simulink model "MPC_Cotroller_ahi"  (R2023a)
settings: Solver=FixedStepAuto  StartTime=0.0  StopTime=10  FixedStep=0.02  RelTol=1e-3
settings Model: Creator=NEW  LastModifiedBy=NEW
settings DebuggingCC: UnderSpecifiedDimensionMsg=warning

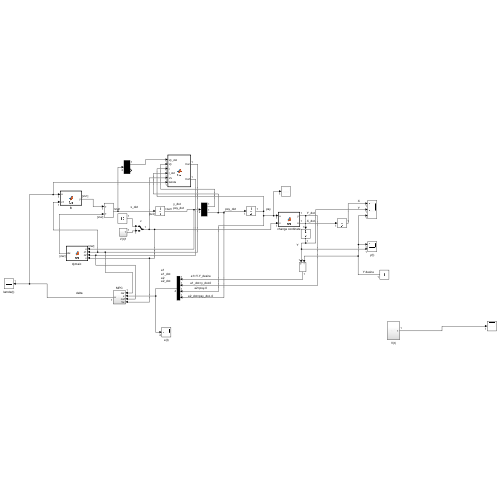
[thumbnail: Simulink's stored preview of the top-level diagram]
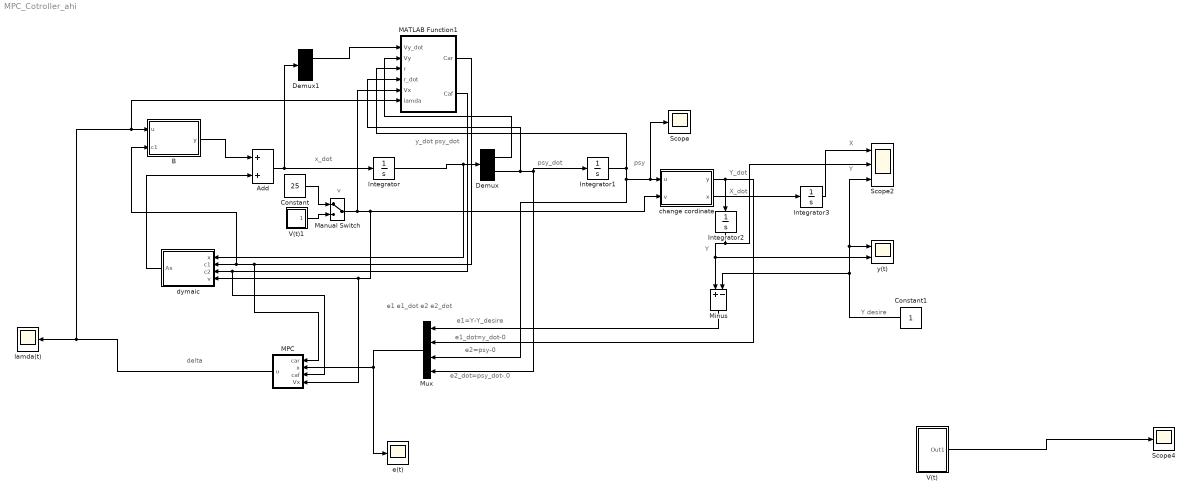
== system MPC_Cotroller_ahi ==
  note: X
  note: X_dot
  note: delta
  note: v
  note: e1
      | e1_dot
      | e2
      | e2_dot
  note: e2_dot=psy_dot-.0
  note: e2=psy-0
  note: e1_dot=y_dot-0
  note: e1=Y-Y_desire
  note: Y desire
  note: Y
  note: Y_dot
  note: psy
  note: psy_dot
  note: y_dot
      | psy_dot
  note: x_dot
  note: Y
  Add : Sum
  B : MATLAB Function  TreatAsAtomicUnit=on
  Constant : Constant  Value=25
  Constant1 : Constant
  Demux : Demux  Outputs=2
  Demux1 : Demux  Outputs=2
  Integrator{,1..3} (4 alike) : Integrator
  MATLAB Function1 : MATLAB Function  TreatAsAtomicUnit=on
  MPC : Subsystem
  Manual Switch : ManualSwitch
  Minus : Sum  Inputs=+-
  Mux : Mux
  Scope : Scope
  Scope2 : Scope  NumInputPorts=3
  Scope4 : Scope
  V(t) : Subsystem
  V(t)1 : Subsystem
  change cordinate : MATLAB Function  TreatAsAtomicUnit=on
  "dymaic " : MATLAB Function  TreatAsAtomicUnit=on
  e(t) : Scope
  lamda(t) : Scope
  y(t) : Scope  NumInputPorts=2
  wires:
  Integrator/1 -> "dymaic "/1(x), Demux/1
  "dymaic "/1(Ax) -> Add/2
  Integrator1/1 -> Mux/3, Scope/1, change cordinate/1(u), MATLAB Function1/3(r)
  Demux/2 -> MATLAB Function1/4(r_dot), Mux/4, Integrator1/1
  change cordinate/1(y) -> Integrator2/1, Mux/2
  Integrator2/1 -> y(t)/2, Minus/1, Scope2/2
  Minus/1 -> Mux/1
  Mux/1 -> e(t)/1, MPC/2(x)
  MPC/1(u) -> MATLAB Function1/6(lamda), B/1(u), lamda(t)/1
  B/1(y) -> Add/1
  Manual Switch/1 -> MATLAB Function1/5(Vx), "dymaic "/4(v), MPC/4(Vx), change cordinate/2(v)
  V(t)/1(Out1) -> Scope4/1
  Constant/1 -> Manual Switch/1
  V(t)1/1(Out1) -> Manual Switch/2
  Integrator3/1 -> Scope2/1
  change cordinate/2(x) -> Integrator3/1
  Constant1/1 -> Scope2/3, y(t)/1, Minus/2
  Add/1 -> Integrator/1, Demux1/1
  Demux/1 -> MATLAB Function1/2(Vy)
  Demux1/1 -> MATLAB Function1/1(Vy_dot)
  MATLAB Function1/1(Car) -> MPC/1(car), B/2(c1), "dymaic "/2(c1)
  MATLAB Function1/2(Caf) -> MPC/3(caf), "dymaic "/3(c2)

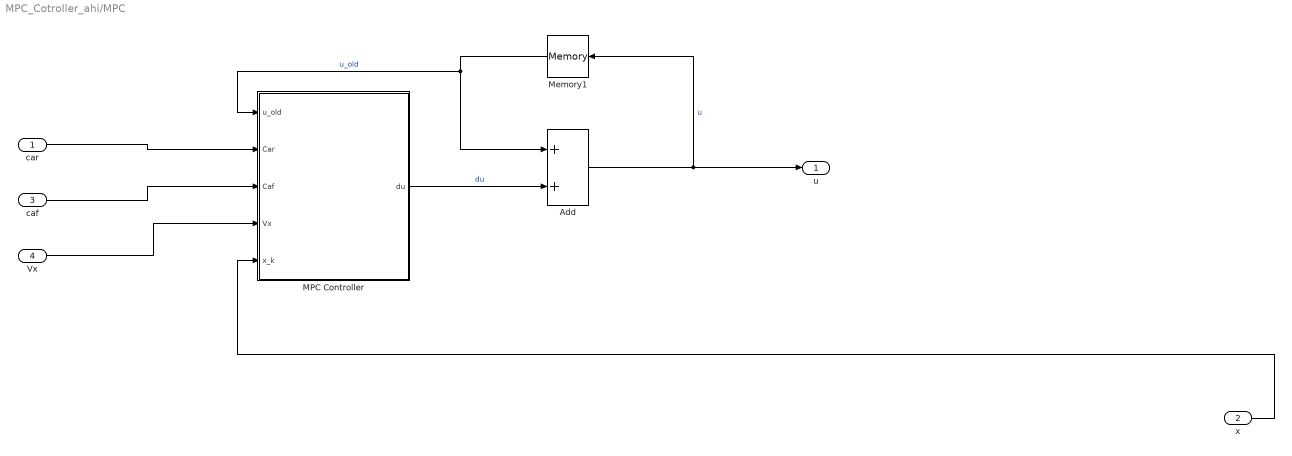
== system MPC_Cotroller_ahi/MPC ==
  car : Inport
  x : Inport  Port=2
  caf : Inport  Port=3
  Vx : Inport  Port=4
  Add : Sum
  MPC Controller : MATLAB Function  TreatAsAtomicUnit=on
  Memory1 : Memory
  u : Outport
  wires:
  Add/1 -> u/1, Memory1/1  "u"
  Memory1/1 -> MPC Controller/1(u_old), Add/1  "u_old"
  MPC Controller/1(du) -> Add/2  "du"
  x/1 -> MPC Controller/5(x_k)
  car/1 -> MPC Controller/2(Car)
  caf/1 -> MPC Controller/3(Caf)
  Vx/1 -> MPC Controller/4(Vx)

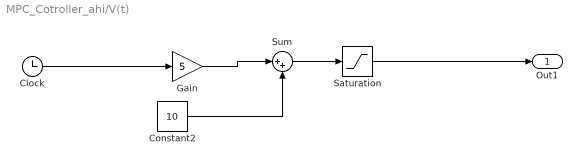
== system MPC_Cotroller_ahi/V(t) ==
  Clock : Clock
  Constant2 : Constant  Value=10
  Gain : Gain  Gain=5
  Saturation : Saturate  UpperLimit=30  LowerLimit=10
  Sum : Sum  Inputs=|++
  Out1 : Outport
  wires:
  Clock/1 -> Gain/1
  Sum/1 -> Saturation/1
  Saturation/1 -> Out1/1
  Constant2/1 -> Sum/2
  Gain/1 -> Sum/1

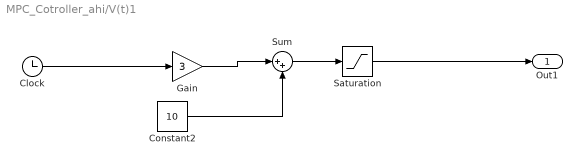
== system MPC_Cotroller_ahi/V(t)1 ==
  Clock : Clock
  Constant2 : Constant  Value=10
  Gain : Gain  Gain=3
  Saturation : Saturate  UpperLimit=30  LowerLimit=10
  Sum : Sum  Inputs=|++
  Out1 : Outport
  wires:
  Clock/1 -> Gain/1
  Sum/1 -> Saturation/1
  Saturation/1 -> Out1/1
  Constant2/1 -> Sum/2
  Gain/1 -> Sum/1

== matlab function MPC_Cotroller_ahi/dymaic  ==
  data: x input; c1 input; Ax output; c2 input; v input
function Ax = fcn(x,c1,c2,v)
%matrix data
m=1734;%[kg]
a=1.422;%[m]
b=1.303;%[m]
I_z=1900;%[kg/m^2]
A_11=-(c1+c2)/(m*v);
A_12=-(v+(a*c1-b*c2)/(m*v));
A_21=-(a*c1-b*c2)/(I_z*v);
A_22=-(a^2*c1+b^2*c2)/(I_z*v);

A=[A_11,A_12;
    A_21,A_22];
Ax = A*x;

== matlab function MPC_Cotroller_ahi/change cordinate ==
  data: u input; y output; v input; x output
function [y,x]= fcn(u,v)
x=v*cos(u);
y = v*sin(u);

== matlab function MPC_Cotroller_ahi/MPC/MPC Controller ==
  data: u_old input; Car input; Caf input; Vx input; du output; x_k input
function du = fcn(u_old,Car ,Caf,Vx, x_k)

du=0; % set output dimentions

%% 1. System Model (function of Vx)
m=1734; Iz=1900;
lr=1.422; lf=1.303; lh=7;


%%% State Space model
A_22=-2*(Caf+Car)/(m*Vx);
A_23= 2*(Caf+Car)/m;
A_24=-2*(Caf*lf-Car*lr)/(m*Vx);
A_42=-2*(Caf*lf-Car*lr)/(Iz*Vx);
A_43= 2*(Caf*lf-Car*lr)/Iz;
A_44=-2*(-Caf*((lf)^2)+Car*((lr)^2))/(Iz*Vx);

B1_2=2*Caf/m;
B1_4=2*Caf*lf/Iz;

A=[0 1 0 0; 0 A_22 A_23 A_24; 0 0 0 1; 0 A_42 A_43 A_44];
B1=[0; B1_2; 0; B1_4];
C=[1 0 0 0; 0 0 1 0];

%% 2. Discretization
Ts=0.02;     % Sampling time [s]
Ad=eye(4)+A*Ts;
B1d=B1*Ts;
Cd=C;

%% 3. Control Problem Parameters
Hp=10;  % Prediction horizon
Hu=2;  % Control Horizon
diagQ=[5 2];  % Weights on output tracking errors
R=1;  % Weights on control inputs rate
U_bond=40*pi/180;  % Control input bound (absolute value)
s_k=[0; 0]; % Set point (zero for regulation)

%% 4. Reference Trajectory convergence rate
Tol_ref=0.05;
Tref=-Ts*Hp/log(Tol_ref);

%% 5. Prediction

% Calculation for i=1
REF=[s_k-exp(-(Ts/Tref))*(s_k-Cd*x_k)];
PSI=[Cd*Ad];
Y=[Cd*B1d];
THETA=[Cd*B1d [0; 0]];
diagQ_=diagQ;

% Calculation for i>1
for i=2:Hp   
    REF=[REF; s_k-exp(-(Ts*i/Tref))*(s_k-Cd*x_k)];
    PSI=[PSI; Cd*(Ad^i)];
    Y=[Y; Cd*polyvalm(ones(1,i),Ad)*B1d];
    THETA=[THETA; Cd*polyvalm(ones(1,i),Ad)*B1d Cd*polyvalm(ones(1,i-1),Ad)*B1d];
    diagQ_=[diagQ_ diagQ];
end

Q_=diag(diagQ_)
R_=diag([R,R]);

Y_free=PSI*x_k+Y*u_old;
EPS=Y_free-REF;

% 4. Quadratic programing (QP) optimization

H_QP=2*(THETA'*Q_*THETA+R_);
f_QP=2*EPS'*Q_*THETA;

A_QP=[1 0;-1 0;1 1;-1 -1];
b_QP=[1; 1; 1; 1]*U_bond+[-1; 1; -1; 1]*u_old;

coder.extrinsic('quadprog');
du_optimal=quadprog(H_QP, f_QP, A_QP, b_QP);
du=du_optimal(1);

== matlab function MPC_Cotroller_ahi/B ==
  data: u input; y output; c1 input
function y = fcn(u,c1)
a=1.422; %[m]
i_z=1900;
m=1734;%[kg]
B1=2*c1/m;
B2=(2*c1*a)/i_z;
B=[B1;B2];
y = B*u;

== matlab function MPC_Cotroller_ahi/MATLAB Function1 ==
  data: Vy_dot input; Car output; Caf output; Vy input; r input; r_dot input; Vx input; lamda input
function [Car,Caf]= fcn(Vy_dot,Vy,r,r_dot,Vx,lamda)
a=1.422;
b=1.303;
m=1734;
l=a+b;
i_zz=1900;
Caf = ((b*Vy_dot*m+b*r*m*Vx+i_zz*r_dot)/l)/((-Vy-r*a+lamda*Vx)/Vx);
Car=((a*r*m*Vx+a*Vy_dot*a*m-i_zz*r_dot)/l)/((r*b-Vy)/Vx);
